simulink model "PMSM_DemoBackup"  (R2020a)
settings: Solver=FixedStepDiscrete  StartTime=0.0  StopTime=Inf  FixedStep=1000e-6  RelTol=1e-3  EnableMultiTasking=on
PreLoadFcn:
  | run('PMSM_Demo_ini.m');
PostLoadFcn:
  | , if any(exist('dsrtsu_mdlpostloadfcn', 'file') ~= 0), dsrtsu_mdlpostloadfcn('Execute', bdroot); end,
InitFcn:
  | , if any(exist('rtifpga_mdlclblib', 'file') ~= 0), rtifpga_mdlclblib('Init', bdroot); end,
undefined symbols (not defined in the file): clock, Const_Id_Fieldweakening, Const_Ld_Stator, Const_Lq_Stator, Const_PolePairs, Const_Psi, Newton, PMSM_Ctrl_Ctrl_mode_SW, PMSM_Ctrl_fRS_Set, PMSM_Ctrl_i_d_Set, PMSM_Ctrl_i_d_Stroke, PMSM_Ctrl_i_q_Set, PMSM_Ctrl_i_q_Stroke, PMSM_Ctrl_Ki_id, PMSM_Ctrl_Ki_iq, PMSM_Ctrl_Ki_n, PMSM_Ctrl_Kp_id, PMSM_Ctrl_Kp_iq, PMSM_Ctrl_Kp_n, PMSM_Ctrl_Limit_iq, PMSM_Ctrl_load_torque, PMSM_Ctrl_n_Limit, PMSM_Ctrl_n_Set, PMSM_Ctrl_n_Stroke, PMSM_Ctrl_Pos_Src, PMSM_Ctrl_TF_Id, PMSM_Ctrl_TF_Iq, PMSM_Ctrl_TF_n, PMSM_Ctrl_theta_offset, PMSM_Ctrl_v_d_Set, PMSM_Ctrl_V_DCLink_Limit, PMSM_Ctrl_v_q_Set, PMSM_Ctrl_Vel_Src, Raphson, rpm_to_rad, s, SW_Fieldweakening, T_PWM
libraries: simulink x37, rti1202lib_adc_class1 x8, dsextras x4, rtiemclib x4, rti1202lib_dio_class1 x3, ASM_ElectricComponents_lib x2, ASM_Utils_lib x1, rti1202lib_base x1
(part 3 of 4)

== system PMSM_DemoBackup/Control/Input/check_inc_valid ==
  note: As long as the encoder has
      | not detected an index signal
      | it's signals are not valid. For this
      | time the hall signals has to be used
  inc_elec_pos : Inport
  hall_pos : Inport  Port=2
  inc_valid : Inport  Port=3
  Switch : Switch  Threshold=0.5
  pos_out : Outport  VectorParamsAs1DForOutWhenUnconnected=off
  wires:
  inc_elec_pos/1 -> Switch/1
  inc_valid/1 -> Switch/2
  Switch/1 -> pos_out/1
  hall_pos/1 -> Switch/3

== system PMSM_DemoBackup/Control/Input/dummy_hall_signals ==
  Ground1 : Ground
  hall_freqbased_vel : Outport  VectorParamsAs1DForOutWhenUnconnected=off
  wires:
  Ground1/1 -> hall_freqbased_vel/1  "hall_freqbased_vel"

== system PMSM_DemoBackup/Control/Input/mech2elec ==
  elec. Angle Offset : Inport
  mech angle : Inport  Port=2
  Constant4 : Constant  Value=360
  Gain3 : Gain  Gain=4
  Math Function : Math  Operator=mod  SignedPower=on  SaturateOnIntegerOverflow=on
  Sum : Sum  Inputs=|++
  elec angle : Outport  VectorParamsAs1DForOutWhenUnconnected=off
  wires:
  elec. Angle Offset/1 -> Sum/1
  Gain3/1 -> Sum/2
  Sum/1 -> Math Function/1
  Math Function/1 -> elec angle/1  "Inc_elec_pos"
  Constant4/1 -> Math Function/2
  mech angle/1 -> Gain3/1

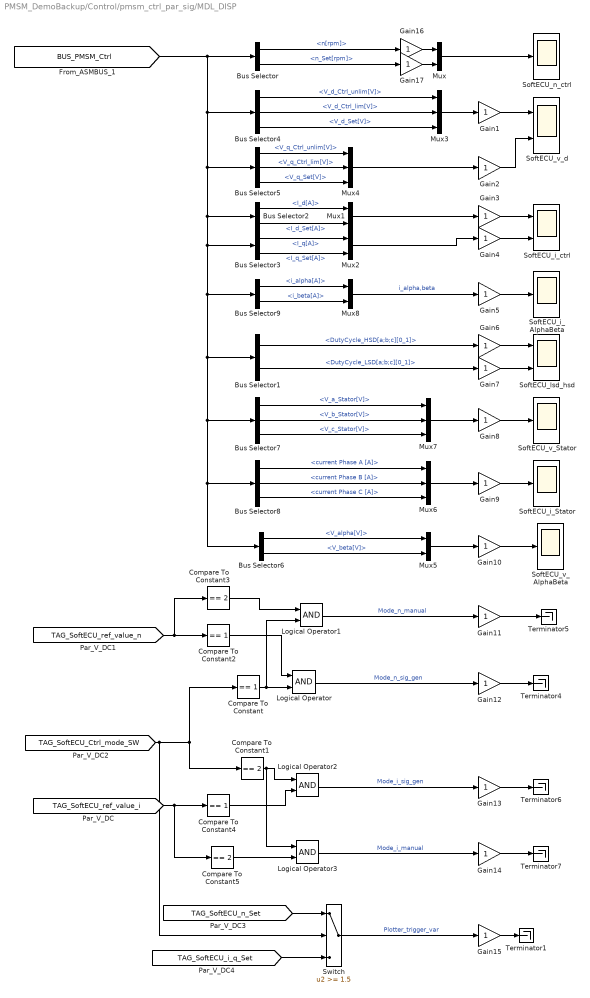
== system PMSM_DemoBackup/Control/pmsm_ctrl_par_sig/MDL_DISP ==
  Bus Selector : BusSelector  OutputSignals=PMSM_Ctrl.PMSM_CONTROLLER.ASMSignalBus_Speed_Controller.n[rpm],PMSM_Ctrl.PMSM_CONTROLLER.ASMSignalBus_Speed_Controller.n_Set[rpm]
  Bus Selector1 : BusSelector  OutputSignals=PMSM_Ctrl.SPACE_VECTOR_MODULATOR.DutyCycle_HSD[a;b;c][0_1],PMSM_Ctrl.SPACE_VECTOR_MODULATOR.DutyCycle_LSD[a;b;c][0_1]
  Bus Selector2 : BusSelector  OutputSignals=PMSM_Ctrl.PMSM_CONTROLLER.ASMSignalBus_Current_Controller.I_d[A],PMSM_Ctrl.PMSM_CONTROLLER.ASMSignalBus_Current_Controller.I_d_Set[A]
  Bus Selector3 : BusSelector  OutputSignals=PMSM_Ctrl.PMSM_CONTROLLER.ASMSignalBus_Current_Controller.I_q[A],PMSM_Ctrl.PMSM_CONTROLLER.ASMSignalBus_Current_Controller.I_q_Set[A]
  Bus Selector4 : BusSelector  OutputSignals=PMSM_Ctrl.PMSM_CONTROLLER.ASMSignalBus_Current_Controller.V_d_Ctrl_unlim[V],PMSM_Ctrl.PMSM_CONTROLLER.ASMSignalBus_Current_Controller.V_d_Ctrl_lim[V],PMSM_Ctrl.PMSM_CONTROLLER.ASMSignalBus_Current_Controller.V_d_Set[V]
  Bus Selector5 : BusSelector  OutputSignals=PMSM_Ctrl.PMSM_CONTROLLER.ASMSignalBus_Current_Controller.V_q_Ctrl_unlim[V],PMSM_Ctrl.PMSM_CONTROLLER.ASMSignalBus_Current_Controller.V_q_Ctrl_lim[V],PMSM_Ctrl.PMSM_CONTROLLER.ASMSignalBus_Current_Controller.V_q_Set[V]
  Bus Selector6 : BusSelector  OutputSignals=PMSM_Ctrl.PMSM_CONTROLLER.V_alpha[V],PMSM_Ctrl.PMSM_CONTROLLER.V_beta[V]
  Bus Selector7 : BusSelector  OutputSignals=PMSM_Ctrl.PMSM_CONTROLLER.v_Stator[a;b;c][V].V_a_Stator[V],PMSM_Ctrl.PMSM_CONTROLLER.v_Stator[a;b;c][V].V_b_Stator[V],PMSM_Ctrl.PMSM_CONTROLLER.v_Stator[a;b;c][V].V_c_Stator[V]
  Bus Selector8 : BusSelector  OutputSignals=PMSM_Ctrl.PMSM_CONTROLLER.i_Stator[a;b;c][A].current Phase A [A],PMSM_Ctrl.PMSM_CONTROLLER.i_Stator[a;b;c][A].current Phase B [A],PMSM_Ctrl.PMSM_CONTROLLER.i_Stator[a;b;c][A].current Phase C [A]
  Bus Selector9 : BusSelector  OutputSignals=PMSM_Ctrl.PMSM_CONTROLLER.ASMSignalBus_Current_Controller.i_alpha[A],PMSM_Ctrl.PMSM_CONTROLLER.ASMSignalBus_Current_Controller.i_beta[A]
  Compare To Constant : simulink/Logic and Bit Operations/Compare To Constant  relop===  const=1  OutDataTypeStr=uint8  ZeroCross=off
  Compare To Constant1 : simulink/Logic and Bit Operations/Compare To Constant  relop===  const=2  OutDataTypeStr=uint8  ZeroCross=off
  Compare To Constant2 : simulink/Logic and Bit Operations/Compare To Constant  relop===  const=1  OutDataTypeStr=uint8  ZeroCross=off
  Compare To Constant3 : simulink/Logic and Bit Operations/Compare To Constant  relop===  const=2  OutDataTypeStr=uint8  ZeroCross=off
  Compare To Constant4 : simulink/Logic and Bit Operations/Compare To Constant  relop===  const=1  OutDataTypeStr=uint8  ZeroCross=off
  Compare To Constant5 : simulink/Logic and Bit Operations/Compare To Constant  relop===  const=2  OutDataTypeStr=uint8  ZeroCross=off
  Gain{1..17} (17 alike) : Gain
  Logical Operator{,1..3} (4 alike) : Logic  AllPortsSameDT=off  OutDataTypeStr=boolean
  Mux{,1..2,5,8} (5 alike) : Mux  Inputs=2
  Mux{3..4,6..7} (4 alike) : Mux  Inputs=3
  SoftECU_i_AlphaBeta : Scope
  SoftECU_i_Stator : Scope
  SoftECU_i_ctrl : Scope  NumInputPorts=2
  SoftECU_lsd_hsd : Scope  NumInputPorts=2
  SoftECU_n_ctrl : Scope
  SoftECU_v_AlphaBeta : Scope
  SoftECU_v_Stator : Scope
  SoftECU_v_d : Scope  NumInputPorts=2
  Switch : Switch  Threshold=1.5
  Terminator{1,4..7} (5 alike) : Terminator
  wires:
  Bus Selector5/3 -> Mux4/3  "<V_q_Set[V]>"
  Bus Selector4/3 -> Mux3/3  "<V_d_Set[V]>"
  Mux2/1 -> Gain4/1
  Mux4/1 -> Gain2/1
  [BUS_PMSM_Ctrl] -> Bus Selector/1, Bus Selector4/1, Bus Selector3/1, Bus Selector7/1, Bus Selector8/1, Bus Selector6/1, Bus Selector1/1, Bus Selector9/1, Bus Selector2/1, Bus Selector5/1
  Bus Selector/1 -> Gain16/1  "<n[rpm]>"
  Bus Selector/2 -> Gain17/1  "<n_Set[rpm]>"
  Bus Selector1/1 -> Gain6/1  "<DutyCycle_HSD[a;b;c][0_1]>"
  Bus Selector1/2 -> Gain7/1  "<DutyCycle_LSD[a;b;c][0_1]>"
  Bus Selector2/1 -> Mux1/1  "<I_d[A]>"
  Bus Selector2/2 -> Mux1/2  "<I_d_Set[A]>"
  Mux1/1 -> Gain3/1
  Bus Selector3/1 -> Mux2/1  "<I_q[A]>"
  Bus Selector3/2 -> Mux2/2  "<I_q_Set[A]>"
  Bus Selector4/1 -> Mux3/1  "<V_d_Ctrl_unlim[V]>"
  Bus Selector4/2 -> Mux3/2  "<V_d_Ctrl_lim[V]>"
  Mux3/1 -> Gain1/1
  Bus Selector5/1 -> Mux4/1  "<V_q_Ctrl_unlim[V]>"
  Bus Selector5/2 -> Mux4/2  "<V_q_Ctrl_lim[V]>"
  Bus Selector6/1 -> Mux5/1  "<V_alpha[V]>"
  Bus Selector6/2 -> Mux5/2  "<V_beta[V]>"
  Mux5/1 -> Gain10/1
  Bus Selector8/1 -> Mux6/1  "<current Phase A [A]>"
  Bus Selector8/2 -> Mux6/2  "<current Phase B [A]>"
  Bus Selector8/3 -> Mux6/3  "<current Phase C [A]>"
  Mux6/1 -> Gain9/1
  Bus Selector7/1 -> Mux7/1  "<V_a_Stator[V]>"
  Bus Selector7/2 -> Mux7/2  "<V_b_Stator[V]>"
  Bus Selector7/3 -> Mux7/3  "<V_c_Stator[V]>"
  Mux7/1 -> Gain8/1
  Bus Selector9/1 -> Mux8/1  "<i_alpha[A]>"
  Bus Selector9/2 -> Mux8/2  "<i_beta[A]>"
  Mux8/1 -> Gain5/1  "i_alpha,beta"
  [TAG_SoftECU_Ctrl_mode_SW] -> Compare To Constant/1, Compare To Constant1/1, Switch/2
  [TAG_SoftECU_ref_value_n] -> Compare To Constant2/1, Compare To Constant3/1
  Compare To Constant/1 -> Logical Operator/2, Logical Operator1/2
  Logical Operator/1 -> Gain12/1  "Mode_n_sig_gen"
  Compare To Constant2/1 -> Logical Operator/1
  Logical Operator1/1 -> Gain11/1  "Mode_n_manual"
  Compare To Constant3/1 -> Logical Operator1/1
  Compare To Constant1/1 -> Logical Operator2/1, Logical Operator3/1
  [TAG_SoftECU_ref_value_i] -> Compare To Constant4/1, Compare To Constant5/1
  Compare To Constant4/1 -> Logical Operator2/2
  Logical Operator2/1 -> Gain13/1  "Mode_i_sig_gen"
  Compare To Constant5/1 -> Logical Operator3/2
  Logical Operator3/1 -> Gain14/1  "Mode_i_manual"
  [TAG_SoftECU_n_Set] -> Switch/1
  [TAG_SoftECU_i_q_Set] -> Switch/3
  Switch/1 -> Gain15/1  "Plotter_trigger_var"
  Mux/1 -> SoftECU_n_ctrl/1
  Gain1/1 -> SoftECU_v_d/1
  Gain2/1 -> SoftECU_v_d/2
  Gain3/1 -> SoftECU_i_ctrl/1
  Gain4/1 -> SoftECU_i_ctrl/2
  Gain5/1 -> SoftECU_i_AlphaBeta/1
  Gain6/1 -> SoftECU_lsd_hsd/1
  Gain7/1 -> SoftECU_lsd_hsd/2
  Gain8/1 -> SoftECU_v_Stator/1
  Gain9/1 -> SoftECU_i_Stator/1
  Gain10/1 -> SoftECU_v_AlphaBeta/1
  Gain11/1 -> Terminator5/1
  Gain12/1 -> Terminator4/1
  Gain13/1 -> Terminator6/1
  Gain14/1 -> Terminator7/1
  Gain15/1 -> Terminator1/1
  Gain16/1 -> Mux/1
  Gain17/1 -> Mux/2

== system PMSM_DemoBackup/Control/pmsm_ctrl_par_sig/MDL_DISP_INPUT ==
  Bus Selector2 : BusSelector  OutputSignals=PMSM_in.Hall_Signals.hall_elec_pos,PMSM_in.Hall_Signals.hall_freqbased_vel,PMSM_in.Hall_Signals.hall_signals
  Bus Selector3 : BusSelector  OutputSignals=PMSM_in.ADC_Voltages
  Bus Selector4 : BusSelector  OutputSignals=PMSM_in.Inc_Signals.Inc_mech_pos,PMSM_in.Inc_Signals.Inc_elec_pos,PMSM_in.Inc_Signals.inc_derivative_vel
  Mux1 : Mux  Inputs=3
  Mux2 : Mux  Inputs=1
  Mux3 : Mux  Inputs=3
  Terminator1 : Terminator
  Terminator2 : Terminator
  Terminator3 : Terminator
  wires:
  [BUS_Inputs] -> Bus Selector4/1, Bus Selector2/1, Bus Selector3/1
  Mux2/1 -> Terminator3/1
  Bus Selector2/1 -> Mux1/1  "<hall_elec_pos>"
  Mux1/1 -> Terminator2/1
  Bus Selector3/1 -> Mux2/1  "<ADC_Voltages>"
  Bus Selector2/2 -> Mux1/2  "<hall_freqbased_vel>"
  Bus Selector4/1 -> Mux3/1  "<Inc_mech_pos>"
  Bus Selector4/2 -> Mux3/2  "<Inc_elec_pos>"
  Mux3/1 -> Terminator1/1
  Bus Selector2/3 -> Mux1/3  "<hall_signals>"
  Bus Selector4/3 -> Mux3/3  "<inc_derivative_vel>"

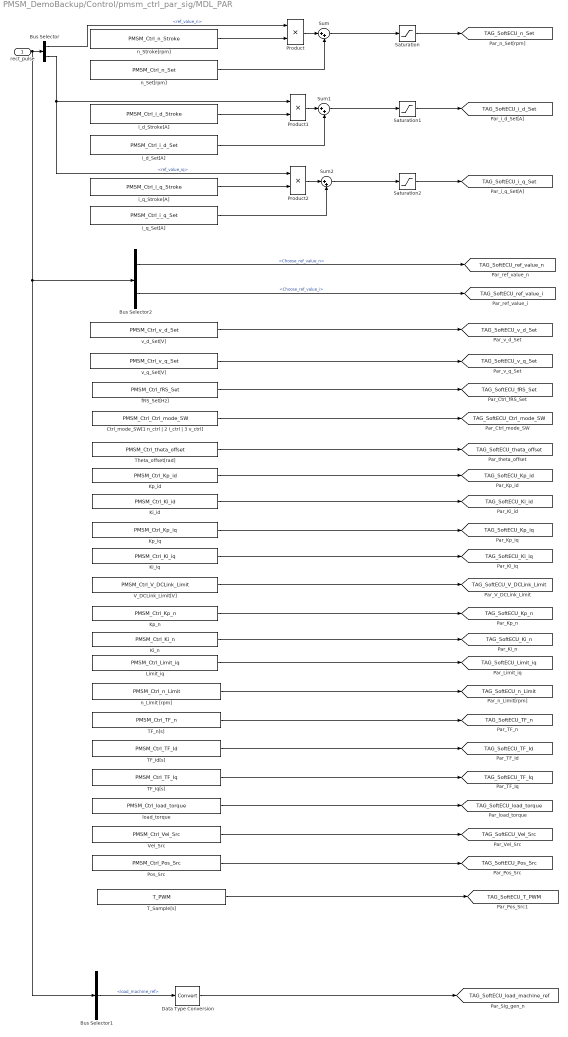
== system PMSM_DemoBackup/Control/pmsm_ctrl_par_sig/MDL_PAR ==
  rect_pulse : Inport
  Bus Selector : BusSelector  OutputSignals=ref_value_n,ref_value_iq
  Bus Selector1 : BusSelector  OutputSignals=load_machine_ref
  Bus Selector2 : BusSelector  OutputSignals=Choose_ref_value_n,Choose_ref_value_i
  Ctrl_mode_SW[1 n_ctrl | 2 i_ctrl | 3 v_ctrl] : Constant  Value=PMSM_Ctrl_Ctrl_mode_SW
  Data Type Conversion : DataTypeConversion
  Ki_id : Constant  Value=PMSM_Ctrl_Ki_id
  Ki_iq : Constant  Value=PMSM_Ctrl_Ki_iq
  Ki_n : Constant  Value=PMSM_Ctrl_Ki_n
  Kp_id : Constant  Value=PMSM_Ctrl_Kp_id
  Kp_iq : Constant  Value=PMSM_Ctrl_Kp_iq
  Kp_n : Constant  Value=PMSM_Ctrl_Kp_n
  Limit_iq : Constant  Value=PMSM_Ctrl_Limit_iq
  Pos_Src : Constant  Value=PMSM_Ctrl_Pos_Src
  Product : Product  RndMeth=Zero
  Product1 : Product  RndMeth=Zero
  Product2 : Product  RndMeth=Zero
  Saturation : Saturate  UpperLimit=1200  LowerLimit=-1200
  Saturation1 : Saturate  UpperLimit=6  LowerLimit=-6
  Saturation2 : Saturate  UpperLimit=6  LowerLimit=-6
  Sum : Sum  Inputs=|++
  Sum1 : Sum  Inputs=|++
  Sum2 : Sum  Inputs=|++
  TF_Id[s] : Constant  Value=PMSM_Ctrl_TF_Id
  TF_Iq[s] : Constant  Value=PMSM_Ctrl_TF_Iq
  TF_n[s] : Constant  Value=PMSM_Ctrl_TF_n
  T_Sample[s] : Constant  Value=T_PWM
  Theta_offset[rad] : Constant  Value=PMSM_Ctrl_theta_offset
  V_DCLink_Limit[V] : Constant  Value=PMSM_Ctrl_V_DCLink_Limit
  Vel_Src : Constant  Value=PMSM_Ctrl_Vel_Src
  fRS_Set[Hz] : Constant  Value=PMSM_Ctrl_fRS_Set
  i_d_Set[A] : Constant  Value=PMSM_Ctrl_i_d_Set
  i_d_Stroke[A] : Constant  Value=PMSM_Ctrl_i_d_Stroke
  i_q_Set[A] : Constant  Value=PMSM_Ctrl_i_q_Set
  i_q_Stroke[A] : Constant  Value=PMSM_Ctrl_i_q_Stroke
  load_torque : Constant  Value=PMSM_Ctrl_load_torque
  n_Limit [rpm] : Constant  Value=PMSM_Ctrl_n_Limit
  n_Set[rpm] : Constant  Value=PMSM_Ctrl_n_Set
  n_Stroke[rpm] : Constant  Value=PMSM_Ctrl_n_Stroke
  v_d_Set[V] : Constant  Value=PMSM_Ctrl_v_d_Set
  v_q_Set[V] : Constant  Value=PMSM_Ctrl_v_q_Set
  tag scope: TAG_SoftECU_Ctrl_mode_SW=global, TAG_SoftECU_Ki_id=global, TAG_SoftECU_Ki_iq=global, TAG_SoftECU_Ki_n=global, TAG_SoftECU_Kp_id=global, TAG_SoftECU_Kp_iq=global, TAG_SoftECU_Kp_n=global, TAG_SoftECU_Limit_iq=global, TAG_SoftECU_Pos_Src=global, TAG_SoftECU_TF_Id=global, TAG_SoftECU_TF_Iq=global, TAG_SoftECU_TF_n=global, TAG_SoftECU_T_PWM=global, TAG_SoftECU_V_DCLink_Limit=global, TAG_SoftECU_Vel_Src=global, TAG_SoftECU_fRS_Set=global, TAG_SoftECU_i_d_Set=global, TAG_SoftECU_i_q_Set=global, TAG_SoftECU_load_machine_ref=global, TAG_SoftECU_load_torque=global, TAG_SoftECU_n_Limit=global, TAG_SoftECU_n_Set=global, TAG_SoftECU_ref_value_i=global, TAG_SoftECU_ref_value_n=global, TAG_SoftECU_theta_offset=global, TAG_SoftECU_v_d_Set=global, TAG_SoftECU_v_q_Set=global
  wires:
  Limit_iq/1 -> [TAG_SoftECU_Limit_iq]
  Ki_n/1 -> [TAG_SoftECU_Ki_n]
  Kp_n/1 -> [TAG_SoftECU_Kp_n]
  V_DCLink_Limit[V]/1 -> [TAG_SoftECU_V_DCLink_Limit]
  Ki_iq/1 -> [TAG_SoftECU_Ki_iq]
  Kp_iq/1 -> [TAG_SoftECU_Kp_iq]
  Ki_id/1 -> [TAG_SoftECU_Ki_id]
  Kp_id/1 -> [TAG_SoftECU_Kp_id]
  Theta_offset[rad]/1 -> [TAG_SoftECU_theta_offset]
  v_d_Set[V]/1 -> [TAG_SoftECU_v_d_Set]
  Ctrl_mode_SW[1 n_ctrl | 2 i_ctrl | 3 v_ctrl]/1 -> [TAG_SoftECU_Ctrl_mode_SW]
  fRS_Set[Hz]/1 -> [TAG_SoftECU_fRS_Set]
  v_q_Set[V]/1 -> [TAG_SoftECU_v_q_Set]
  n_Limit [rpm]/1 -> [TAG_SoftECU_n_Limit]
  TF_n[s]/1 -> [TAG_SoftECU_TF_n]
  TF_Id[s]/1 -> [TAG_SoftECU_TF_Id]
  TF_Iq[s]/1 -> [TAG_SoftECU_TF_Iq]
  load_torque/1 -> [TAG_SoftECU_load_torque]
  Sum/1 -> Saturation/1
  Product/1 -> Sum/1
  Product1/1 -> Sum1/1
  Sum1/1 -> Saturation1/1
  Product2/1 -> Sum2/1
  Sum2/1 -> Saturation2/1
  n_Set[rpm]/1 -> Sum/2
  i_d_Set[A]/1 -> Sum1/2
  i_q_Set[A]/1 -> Sum2/2
  n_Stroke[rpm]/1 -> Product/2
  i_d_Stroke[A]/1 -> Product1/2
  i_q_Stroke[A]/1 -> Product2/2
  Vel_Src/1 -> [TAG_SoftECU_Vel_Src]
  Pos_Src/1 -> [TAG_SoftECU_Pos_Src]
  T_Sample[s]/1 -> [TAG_SoftECU_T_PWM]
  Saturation/1 -> [TAG_SoftECU_n_Set]
  Saturation1/1 -> [TAG_SoftECU_i_d_Set]
  Saturation2/1 -> [TAG_SoftECU_i_q_Set]
  rect_pulse/1 -> Bus Selector/1, Bus Selector1/1, Bus Selector2/1
  Bus Selector/1 -> Product/1  "<ref_value_n>"
  Bus Selector/2 -> Product1/1, Product2/1  "<ref_value_iq>"
  Bus Selector1/1 -> Data Type Conversion/1  "<load_machine_ref>"
  Bus Selector2/1 -> [TAG_SoftECU_ref_value_n]  "<Choose_ref_value_n>"
  Bus Selector2/2 -> [TAG_SoftECU_ref_value_i]  "<Choose_ref_value_i>"
  Data Type Conversion/1 -> [TAG_SoftECU_load_machine_ref]

== system PMSM_DemoBackup/RTI Data/RTI Data Store/RTI Data Store ==
  RTI Data Store : Subsystem  mask(RTI_DATA_STORE){}
      mask help:
      | RTI Data Store Block. This block is used by RTI to store internal model dependent data. Deleting this block will result in data loss.
      |
      | NEVER DELETE, COPY, OR MODIFY THIS BLOCK!
      mask Help:
      | RTI Data Store Block. This block is used by RTI to store internal model dependent data. Deleting this block will result in data loss.
      | 
      | NEVER DELETE, COPY, OR MODIFY THIS BLOCK!
      mask Display: text(0.5, 0.5, ' ', 'HorizontalAlignment', 'center');

== system PMSM_DemoBackup/Control/Control_load_machine/duty_cycle_2_torque/duty_cycle_2_voltage ==
  In_duty_cycle[0..1] : Inport
  Bus Selector : BusSelector  OutputSignals=ADC_Voltages.Battery_Voltage[V]
  Divide : Product  Inputs=**
  Saturation1 : Saturate  UpperLimit=1  LowerLimit=0
  Out_duty_voltage[V] : Outport  VectorParamsAs1DForOutWhenUnconnected=off
  wires:
  Divide/1 -> Out_duty_voltage[V]/1
  In_duty_cycle[0..1]/1 -> Saturation1/1
  Bus Selector/1 -> Divide/2  "<Battery_Voltage[V]>"
  [BUS_PMSM_IN] -> Bus Selector/1
  Saturation1/1 -> Divide/1

== system PMSM_DemoBackup/Control/Control_load_machine/torque_2_duty_cycle/voltage_2_duty_cycle ==
  In_voltage[V] : Inport
  Bus Selector : BusSelector  OutputSignals=ADC_Voltages.Battery_Voltage[V]
  Divide : Product  Inputs=*/
  Saturation : Saturate  UpperLimit=1  LowerLimit=0
  Out_duty_cycle : Outport  VectorParamsAs1DForOutWhenUnconnected=off
  wires:
  Divide/1 -> Saturation/1
  In_voltage[V]/1 -> Divide/1
  Saturation/1 -> Out_duty_cycle/1
  Bus Selector/1 -> Divide/2  "<Battery_Voltage[V]>"
  [BUS_PMSM_IN] -> Bus Selector/1

== system PMSM_DemoBackup/Control/Control_load_machine/torque_2_duty_cycle1/voltage_2_duty_cycle ==
  In_voltage[V] : Inport
  Bus Selector : BusSelector  OutputSignals=ADC_Voltages.Battery_Voltage[V]
  Divide : Product  Inputs=*/
  Saturation : Saturate  UpperLimit=1  LowerLimit=0
  Out_duty_cycle[0..1] : Outport  VectorParamsAs1DForOutWhenUnconnected=off
  wires:
  [BUS_PMSM_IN] -> Bus Selector/1
  Bus Selector/1 -> Divide/2  "<Battery_Voltage[V]>"
  Saturation/1 -> Out_duty_cycle[0..1]/1
  In_voltage[V]/1 -> Divide/1
  Divide/1 -> Saturation/1

== system PMSM_DemoBackup/Control/Controller/PMSM_CONTROLLER/5x_mean_value ==
  n[rpm] : Inport
  Gain : Gain  Gain=1/5
  Memory{,1..3} (4 alike) : Memory  InheritSampleTime=on
  Sum : Sum  Inputs=+++++
  n_mean[rpm] : Outport  VectorParamsAs1DForOutWhenUnconnected=off
  wires:
  n[rpm]/1 -> Sum/1, Memory/1
  Memory/1 -> Sum/2, Memory1/1
  Memory1/1 -> Sum/3, Memory2/1
  Memory2/1 -> Sum/4, Memory3/1
  Memory3/1 -> Sum/5
  Sum/1 -> Gain/1
  Gain/1 -> n_mean[rpm]/1

== system PMSM_DemoBackup/Control/Controller/PMSM_CONTROLLER/SignalCollector ==
  SignalBus_Speed_Controller : Inport
  V_DCLink[V] : Inport  Port=2
  i_Stator[a;b;c][A] : Inport  Port=3
  SignalBus_Current_Controller : Inport  Port=4
  V_d[V] : Inport  Port=5
  V_q[V] : Inport  Port=6
  V_alpha[V] : Inport  Port=7
  V_beta[V] : Inport  Port=8
  v_Stator[a;b;c][V] : Inport  Port=9
  Bus Creator : BusCreator  Inputs=9
  SignalBus : Outport  VectorParamsAs1DForOutWhenUnconnected=off
  wires:
  SignalBus_Current_Controller/1 -> Bus Creator/2  "ASMSignalBus_Current_Controller"
  SignalBus_Speed_Controller/1 -> Bus Creator/1  "ASMSignalBus_Speed_Controller"
  V_q[V]/1 -> Bus Creator/7  "V_q_Set[V]"
  V_d[V]/1 -> Bus Creator/6  "V_d_Set[V]"
  Bus Creator/1 -> SignalBus/1  "PMSM_CONTROLLER"
  V_DCLink[V]/1 -> Bus Creator/5  "V_DCLink[V]"
  i_Stator[a;b;c][A]/1 -> Bus Creator/3  "i_Stator[a;b;c][A]"
  v_Stator[a;b;c][V]/1 -> Bus Creator/4  "v_Stator[a;b;c][V]"
  V_alpha[V]/1 -> Bus Creator/8  "V_alpha[V]"
  V_beta[V]/1 -> Bus Creator/9  "V_beta[V]"

== system PMSM_DemoBackup/Control/Controller/PMSM_CONTROLLER/Trigger_250us ==
  Counter Limited : simulink/Sources/Counter Limited  uplimit=4  tsamp=-1
  Lookup Table : Lookup_n-D  NumberOfTableDimensions=1  BreakpointsForDimension1=[0,1,2,3,4]  Table=[1,0,0,0,0]  ExtrapMethod=Clip  InputSameDT=on
  trigger : Outport  VectorParamsAs1DForOutWhenUnconnected=off
  wires:
  Counter Limited/1 -> Lookup Table/1
  Lookup Table/1 -> trigger/1

== system PMSM_DemoBackup/Control/Controller/PMSM_CONTROLLER/angle_calculation ==
  n[rpm] : Inport
  eps [rad] : Inport  Port=2
  eps_offset[rad] : Inport  Port=3
  T_Sample[s] : Inport  Port=4
  Const_PolePair[] : Constant  Value=Const_PolePair
  Lim[0...2*pi] : Subsystem
  Product1 : Product  RndMeth=Zero
  Product2 : Product  RndMeth=Zero
  Sum : Sum  Inputs=|++
  Terminator : Terminator
  toRad|s : Gain  Gain=pi/30  SaturateOnIntegerOverflow=on  OutDataTypeStr=Inherit: Same as input  ParamDataTypeStr=Inherit: Same as input
  eps[rad] : Outport  VectorParamsAs1DForOutWhenUnconnected=off
  omega_el[rad|s] : Outport  Port=2  VectorParamsAs1DForOutWhenUnconnected=off
  eps_komp[rad] : Outport  Port=3  VectorParamsAs1DForOutWhenUnconnected=off
  wires:
  n[rpm]/1 -> Product2/1
  T_Sample[s]/1 -> Product1/1
  Product1/1 -> Terminator/1
  toRad|s/1 -> Product1/2, omega_el[rad|s]/1
  Product2/1 -> toRad|s/1
  Const_PolePair[]/1 -> Product2/2
  Lim[0...2*pi]/1(theta_lim) -> eps[rad]/1, eps_komp[rad]/1
  eps [rad]/1 -> Sum/1
  Sum/1 -> Lim[0...2*pi]/1(theta_unlim)
  eps_offset[rad]/1 -> Sum/2

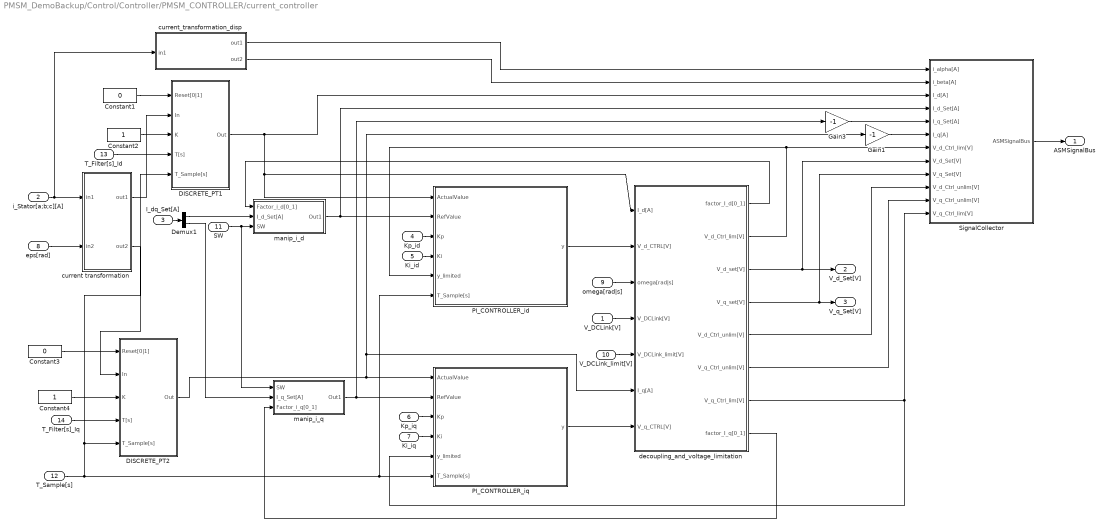
== system PMSM_DemoBackup/Control/Controller/PMSM_CONTROLLER/current_controller ==
  V_DCLink[V] : Inport
  i_Stator[a;b;c][A] : Inport  Port=2
  I_dq_Set[A] : Inport  Port=3
  Kp_id : Inport  Port=4
  Ki_id : Inport  Port=5
  Kp_iq : Inport  Port=6
  Ki_iq : Inport  Port=7
  eps[rad] : Inport  Port=8
  omega[rad|s] : Inport  Port=9
  V_DCLink_limit[V] : Inport  Port=10
  SW : Inport  Port=11
  T_Sample[s] : Inport  Port=12
  T_Filter[s]_Id : Inport  Port=13
  T_Filter[s]_Iq : Inport  Port=14
  Constant1 : Constant  Value=0
  Constant2 : Constant
  Constant3 : Constant  Value=0
  Constant4 : Constant
  DISCRETE_PT1 : Subsystem  mask(DISCRETE_PT1){upper_limit_int=struct('v', 1e300), lower_limit_int=struct('v', -1e300), ASMProperties=struct('Name','DISCRETE_PT1','Version','1.0','Library','ASM_ElectricComponents_lib')}
      mask prompts: upper_limit_int "upper limit (Integrator)"; lower_limit_int "lower limit (Integrator)"
      mask help: (c) Copyright 2007, dSPACE GmbH. All rights reserved.
      mask Help: eval(['asm_modelhelp(gcbh)'])
  DISCRETE_PT2 : Subsystem  mask(DISCRETE_PT1){upper_limit_int=struct('v', 1e300), lower_limit_int=struct('v', -1e300), ASMProperties=struct('Name','DISCRETE_PT1','Version','1.0','Library','ASM_ElectricComponents_lib')}
      mask prompts: upper_limit_int "upper limit (Integrator)"; lower_limit_int "lower limit (Integrator)"
      mask help: (c) Copyright 2007, dSPACE GmbH. All rights reserved.
      mask Help: eval(['asm_modelhelp(gcbh)'])
  Demux1 : Demux  Outputs=2
  Gain1 : Gain  Gain=-1
  Gain3 : Gain  Gain=-1
  PI_CONTROLLER_id : Subsystem  mask(PI_CONTROLLER_EXT_SATURATION){ASMProperties=struct('Name','PI_CONTROLLER_EXT_SATURATION','Version','1.0','Library','ASM_ElectricComponents_lib')}
      mask help: (c) Copyright 2007, dSPACE GmbH. All rights reserved.
  PI_CONTROLLER_iq : Subsystem  mask(PI_CONTROLLER_EXT_SATURATION){ASMProperties=struct('Name','PI_CONTROLLER_EXT_SATURATION','Version','1.0','Library','ASM_ElectricComponents_lib')}
      mask help: (c) Copyright 2007, dSPACE GmbH. All rights reserved.
  SignalCollector : Subsystem
  current transformation : Subsystem  Description=version  mask(ASM_EC_TRANSFORMATION){transformation=abc            -> d/q              (clarke and park transformation), compin=off, compout=on, zerocomp=off, interm=off, cossinvector=off, powrefframe=off, transffactor=1, transffactor_zero=1, ASMProperties=struct('Name','asm_ec_transformation','Version','1.0','Library','ASM_ElectricComponents_lib')}
      mask prompts: compin "Component wise input"; compout "Component wise output"; zerocomp "Zero component"; interm "Intermediat values"; cossinvector "Cos/Sin vector input"; powrefframe "Power-invariant transformation"
      mask help:
      | Clarke and/or Park transformation for three phase electric system.
      |
      | (c) Copyright 2007, dSPACE GmbH. All rights reserved.
      mask init:
      | %asm_ec_clarkparktrans('DYNATRANSF_Config',gcb);
      settings: AttributesFormatString=park/clark transformation
      mask Help: eval(['asm_modelhelp(gcbh)'])
      mask TypeOptions transformation: abc             -> alpha/beta  (clarke transformation) | alpha/beta -> abc              (inverse clarke transformation) | alpha/beta -> d/q              (park transformation) | d/q             -> alpha/beta  (inverse park transformation) | abc            -> d/q              (clarke and park transformation) | d/q            -> abc              (inverse clarke and park transformation)
      mask Callback transformation: asm_ec_clarkparktrans('DYNATRANSF_ConfigDisp',gcb);
      mask Display: plot([1 0],[1 0]);port_label('input',1,'[3]');port_label('input',2,'eps (rad)');port_label('output',1,'d');port_label('output',2,'q');text(0.042857,0.94898,'a,b,c');text(0.89286,0.05102,'');
  current_transformation_disp : Subsystem  Description=version  mask(ASM_EC_TRANSFORMATION){transformation=abc             -> alpha/beta  (clarke transformation), compin=off, compout=on, zerocomp=off, interm=off, cossinvector=off, powrefframe=off, transffactor=1, transffactor_zero=1, ASMProperties=struct('Name','ASM_EC_TRANSFORMATION','Version','1.0','Library','ASM_ElectricComponents_lib')}
      mask prompts: compin "Component wise input"; compout "Component wise output"; zerocomp "Zero component"; interm "Intermediat values"; cossinvector "Cos/Sin vector input"; powrefframe "Power-invariant transformation"
      mask help:
      | Clarke and/or Park transformation for three phase electric system.
      |
      | (c) Copyright 2007, dSPACE GmbH. All rights reserved.
      mask init:
      | %asm_ec_clarkparktrans('DYNATRANSF_Config',gcb);
      settings: AttributesFormatString=clark transformation
      mask Help: eval(['asm_modelhelp(gcbh)'])
      mask TypeOptions transformation: abc             -> alpha/beta  (clarke transformation) | alpha/beta -> abc              (inverse clarke transformation) | alpha/beta -> d/q              (park transformation) | d/q             -> alpha/beta  (inverse park transformation) | abc            -> d/q              (clarke and park transformation) | d/q            -> abc              (inverse clarke and park transformation)
      mask Callback transformation: asm_ec_clarkparktrans('DYNATRANSF_ConfigDisp',gcb);
      mask Display: plot([1 0],[1 0]);port_label('input',1,'[3]');port_label('output',1,'alpha');port_label('output',2,'beta');text(0.022222,0.85849,'a,b,c');text(0.94444,0.14151,'');
  decoupling_and_voltage_limitation : Subsystem
  manip_i_d : Subsystem
  manip_i_q : Subsystem
  ASMSignalBus : Outport  VectorParamsAs1DForOutWhenUnconnected=off
  " V_d_Set[V]" : Outport  Port=2  VectorParamsAs1DForOutWhenUnconnected=off
  " V_q_Set[V]" : Outport  Port=3  VectorParamsAs1DForOutWhenUnconnected=off
  wires:
  eps[rad]/1 -> current transformation/2(in2)
  i_Stator[a;b;c][A]/1 -> current transformation/1(in1), current_transformation_disp/1(in1)
  SW/1 -> manip_i_q/1(SW), manip_i_d/3(SW)
  decoupling_and_voltage_limitation/1(factor_I_d[0_1]) -> manip_i_d/1(Factor_i_d[0_1])
  decoupling_and_voltage_limitation/8(factor_I_q[0_1]) -> manip_i_q/3(Factor_i_q[0_1])
  T_Sample[s]/1 -> PI_CONTROLLER_id/6(T_Sample[s]), PI_CONTROLLER_iq/6(T_Sample[s]), DISCRETE_PT1/5(T_Sample[s]), DISCRETE_PT2/5(T_Sample[s])
  Demux1/1 -> manip_i_d/2(I_d_Set[A])
  Demux1/2 -> manip_i_q/2(I_q_Set[A])
  Ki_iq/1 -> PI_CONTROLLER_iq/4(Ki)
  Kp_iq/1 -> PI_CONTROLLER_iq/3(Kp)
  Ki_id/1 -> PI_CONTROLLER_id/4(Ki)
  Kp_id/1 -> PI_CONTROLLER_id/3(Kp)
  manip_i_q/1(Out1) -> PI_CONTROLLER_iq/2(RefValue), Gain3/1
  I_dq_Set[A]/1 -> Demux1/1
  decoupling_and_voltage_limitation/6(V_q_Ctrl_unlim[V]) -> SignalCollector/11(V_q_Ctrl_unlim[V])
  decoupling_and_voltage_limitation/5(V_d_Ctrl_unlim[V]) -> SignalCollector/10(V_d_Ctrl_unlim[V])
  SignalCollector/1(ASMSignalBus) -> ASMSignalBus/1
  decoupling_and_voltage_limitation/2(V_d_Ctrl_lim[V]) -> PI_CONTROLLER_id/5(y_limited), SignalCollector/7(V_d_Ctrl_lim[V])
  decoupling_and_voltage_limitation/7(V_q_Ctrl_lim[V]) -> PI_CONTROLLER_iq/5(y_limited), SignalCollector/12(V_q_Ctrl_lim[V])
  V_DCLink[V]/1 -> decoupling_and_voltage_limitation/4(V_DCLink[V])
  manip_i_d/1(Out1) -> SignalCollector/4(I_d_Set[A]), PI_CONTROLLER_id/2(RefValue)
  omega[rad|s]/1 -> decoupling_and_voltage_limitation/3(omega[rad|s])
  PI_CONTROLLER_iq/1(y) -> decoupling_and_voltage_limitation/7(V_q_CTRL[V])
  decoupling_and_voltage_limitation/4(V_q_set[V]) -> " V_q_Set[V]"/1, SignalCollector/9(V_q_Set[V])
  decoupling_and_voltage_limitation/3(V_d_set[V]) -> " V_d_Set[V]"/1, SignalCollector/8(V_d_Set[V])
  PI_CONTROLLER_id/1(y) -> decoupling_and_voltage_limitation/2(V_d_CTRL[V])
  V_DCLink_limit[V]/1 -> decoupling_and_voltage_limitation/5(V_DCLink_limit[V])
  T_Filter[s]_Iq/1 -> DISCRETE_PT2/4(T[s])
  Constant3/1 -> DISCRETE_PT2/1(Reset[0|1])
  Constant4/1 -> DISCRETE_PT2/3(K)
  current transformation/2(out2) -> DISCRETE_PT2/2(In)
  DISCRETE_PT2/1(Out) -> PI_CONTROLLER_iq/1(ActualValue), decoupling_and_voltage_limitation/6(I_q[A]), Gain1/1
  DISCRETE_PT1/1(Out) -> SignalCollector/3(I_d[A]), PI_CONTROLLER_id/1(ActualValue), decoupling_and_voltage_limitation/1(I_d[A])
  current transformation/1(out1) -> DISCRETE_PT1/2(In)
  Constant1/1 -> DISCRETE_PT1/1(Reset[0|1])
  Constant2/1 -> DISCRETE_PT1/3(K)
  T_Filter[s]_Id/1 -> DISCRETE_PT1/4(T[s])
  Gain3/1 -> SignalCollector/5(I_q_Set[A])
  Gain1/1 -> SignalCollector/6(I_q[A])
  current_transformation_disp/1(out1) -> SignalCollector/1(i_alpha[A])
  current_transformation_disp/2(out2) -> SignalCollector/2(i_beta[A])

== system PMSM_DemoBackup/Control/Controller/PMSM_CONTROLLER/i_set_source_SW ==
  I_d_Set_2 : Inport
  I_q_Set_2 : Inport  Port=2
  I_q_Set_1 : Inport  Port=3
  Id_Limit : Inport  Port=4
  Iq_Limit : Inport  Port=5
  SW : Inport  Port=6
  Const_Id_Fieldweakening[A] : Constant  Value=Const_Id_Fieldweakening
  Demux : Demux  Outputs=2
  Gain3 : Gain  Gain=-1
  Limit_id_Set : Subsystem
      mask Display: plot([0.15 0.85],[.5 .5],[.5 .5],[0.05 0.95],0.15+0.7*[0 .25 .75 1],0.05+0.9*[.25 .25 .75 .75]);
  Limit_iq_Set : Subsystem
      mask Display: plot([0.15 0.85],[.5 .5],[.5 .5],[0.05 0.95],0.15+0.7*[0 .25 .75 1],0.05+0.9*[.25 .25 .75 .75]);
  Multiport Switch : MultiPortSwitch
  Mux{,1..3} (4 alike) : Mux  Inputs=2
  zero : Constant  Value=0
  I_dq_Set : Outport  VectorParamsAs1DForOutWhenUnconnected=off
  wires:
  zero/1 -> Mux3/2, Mux3/1
  Mux3/1 -> Multiport Switch/4
  Mux2/1 -> Multiport Switch/3
  Mux1/1 -> Multiport Switch/2
  Mux/1 -> I_dq_Set/1
  Iq_Limit/1 -> Limit_iq_Set/2(In2)
  Id_Limit/1 -> Limit_id_Set/2(In2)
  Limit_id_Set/1(Out1) -> Mux/1
  Demux/1 -> Limit_id_Set/1(In1)
  Limit_iq_Set/1(Out1) -> Mux/2
  Demux/2 -> Limit_iq_Set/1(In1)
  Multiport Switch/1 -> Demux/1
  I_q_Set_1/1 -> Mux1/2
  SW/1 -> Multiport Switch/1
  I_d_Set_2/1 -> Mux2/1
  I_q_Set_2/1 -> Gain3/1
  Const_Id_Fieldweakening[A]/1 -> Mux1/1
  Gain3/1 -> Mux2/2

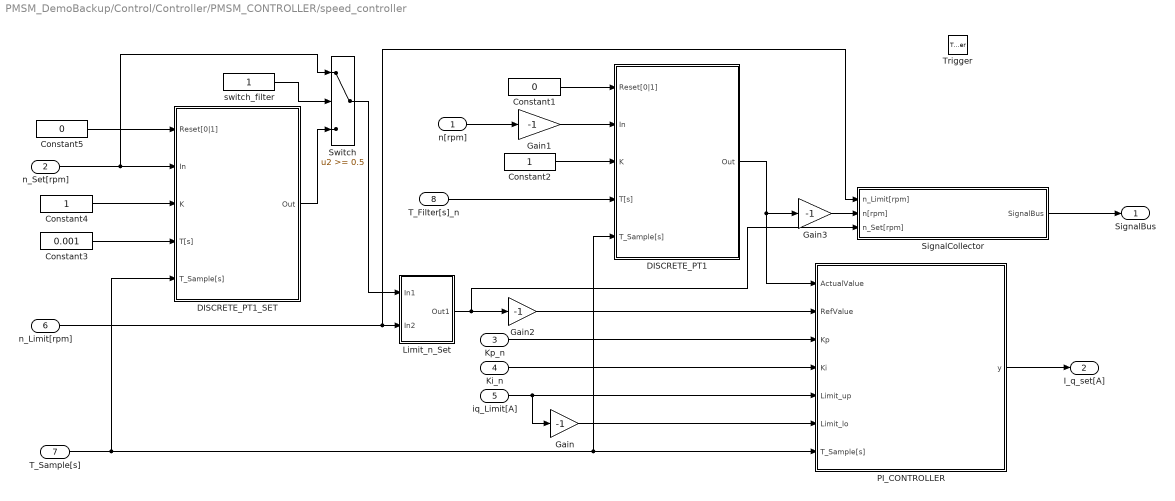
== system PMSM_DemoBackup/Control/Controller/PMSM_CONTROLLER/speed_controller ==
  n[rpm] : Inport
  n_Set[rpm] : Inport  Port=2
  Kp_n : Inport  Port=3
  Ki_n : Inport  Port=4
  iq_Limit[A] : Inport  Port=5
  n_Limit[rpm] : Inport  Port=6
  T_Sample[s] : Inport  Port=7
  T_Filter[s]_n : Inport  Port=8
  Trigger : TriggerPort  VariantControl=Variant
  Constant1 : Constant  Value=0
  Constant2 : Constant
  Constant3 : Constant  Value=0.001
  Constant4 : Constant
  Constant5 : Constant  Value=0
  DISCRETE_PT1 : Subsystem  mask(DISCRETE_PT1){upper_limit_int=struct('v',1e300), lower_limit_int=struct('v', -1e300), ASMProperties=struct('Name','DISCRETE_PT1','Version','1.0','Library','ASM_ElectricComponents_lib')}
      mask prompts: upper_limit_int "upper limit (Integrator)"; lower_limit_int "lower limit (Integrator)"
      mask help: (c) Copyright 2007, dSPACE GmbH. All rights reserved.
      mask Help: eval(['asm_modelhelp(gcbh)'])
  DISCRETE_PT1_SET : Subsystem  mask(DISCRETE_PT1){upper_limit_int=struct('v', 1e300), lower_limit_int=struct('v', -1e300), ASMProperties=struct('Name','DISCRETE_PT1','Version','1.0','Library','ASM_ElectricComponents_lib')}
      mask prompts: upper_limit_int "upper limit (Integrator)"; lower_limit_int "lower limit (Integrator)"
      mask help: (c) Copyright 2007, dSPACE GmbH. All rights reserved.
      mask Help: eval(['asm_modelhelp(gcbh)'])
  Gain{,1..3} (4 alike) : Gain  Gain=-1
  Limit_n_Set : Subsystem
      mask Display: plot([0.15 0.85],[.5 .5],[.5 .5],[0.05 0.95],0.15+0.7*[0 .25 .75 1],0.05+0.9*[.25 .25 .75 .75]);
  PI_CONTROLLER : Subsystem  mask(PI_CONTROLLER){ASMProperties=struct('Name','PI_CONTROLLER','Version','1.0','Library','ASM_ElectricComponents_lib')}
      mask help: (c) Copyright 2007, dSPACE GmbH. All rights reserved.
  SignalCollector : Subsystem
  Switch : Switch  Threshold=0.5
  switch_filter : Constant
  SignalBus : Outport  VectorParamsAs1DForOutWhenUnconnected=off
  I_q_set[A] : Outport  Port=2  VectorParamsAs1DForOutWhenUnconnected=off
  wires:
  SignalCollector/1(SignalBus) -> SignalBus/1
  PI_CONTROLLER/1(y) -> I_q_set[A]/1
  Kp_n/1 -> PI_CONTROLLER/3(Kp)
  Ki_n/1 -> PI_CONTROLLER/4(Ki)
  iq_Limit[A]/1 -> PI_CONTROLLER/5(Limit_up), Gain/1
  Gain/1 -> PI_CONTROLLER/6(Limit_lo)
  T_Sample[s]/1 -> PI_CONTROLLER/7(T_Sample[s]), DISCRETE_PT1/5(T_Sample[s]), DISCRETE_PT1_SET/5(T_Sample[s])
  Limit_n_Set/1(Out1) -> Gain2/1, SignalCollector/3(n_Set[rpm])
  n_Limit[rpm]/1 -> SignalCollector/1(n_Limit[rpm]), Limit_n_Set/2(In2)
  n[rpm]/1 -> Gain1/1
  Gain1/1 -> DISCRETE_PT1/2(In)
  Constant1/1 -> DISCRETE_PT1/1(Reset[0|1])
  Constant2/1 -> DISCRETE_PT1/3(K)
  DISCRETE_PT1/1(Out) -> PI_CONTROLLER/1(ActualValue), Gain3/1
  T_Filter[s]_n/1 -> DISCRETE_PT1/4(T[s])
  Gain2/1 -> PI_CONTROLLER/2(RefValue)
  Gain3/1 -> SignalCollector/2(n[rpm])
  n_Set[rpm]/1 -> DISCRETE_PT1_SET/2(In), Switch/1
  Constant3/1 -> DISCRETE_PT1_SET/4(T[s])
  Constant4/1 -> DISCRETE_PT1_SET/3(K)
  Constant5/1 -> DISCRETE_PT1_SET/1(Reset[0|1])
  DISCRETE_PT1_SET/1(Out) -> Switch/3
  Switch/1 -> Limit_n_Set/1(In1)
  switch_filter/1 -> Switch/2

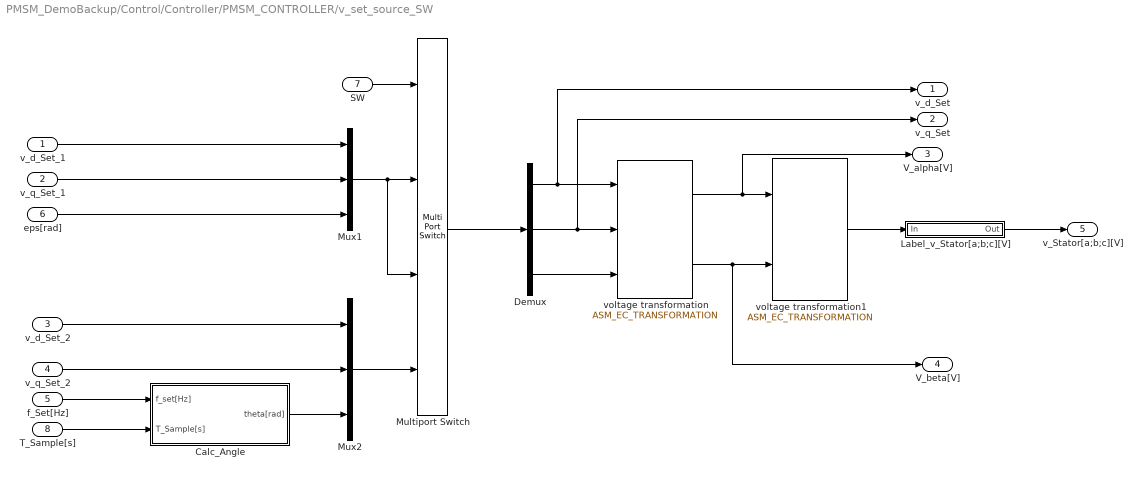
== system PMSM_DemoBackup/Control/Controller/PMSM_CONTROLLER/v_set_source_SW ==
  v_d_Set_1 : Inport
  v_q_Set_1 : Inport  Port=2
  v_d_Set_2 : Inport  Port=3
  v_q_Set_2 : Inport  Port=4
  f_Set[Hz] : Inport  Port=5
  eps[rad] : Inport  Port=6
  SW : Inport  Port=7
  T_Sample[s] : Inport  Port=8
  Calc_Angle : Subsystem
  Demux : Demux  Outputs=3
  Label_v_Stator[a;b;c][V] : Subsystem
  Multiport Switch : MultiPortSwitch
  Mux1 : Mux  Inputs=3
  Mux2 : Mux  Inputs=3
  voltage transformation : ASM_ElectricComponents_lib/Utils/ASM_EC_TRANSFORMATION  Description=version  transformation="d/q             -> alpha/beta  (inverse park transformation)"  compin=on  compout=on  zerocomp=off  interm=off  cossinvector=off  powrefframe=off  transffactor=1  transffactor_zero=1  ASMProperties=struct('Name','asm_ec_transformation','Version','1.0','Library','ASM_ElectricComponents_lib')
      settings: AttributesFormatString=inverse park transformation
  voltage transformation1 : ASM_ElectricComponents_lib/Utils/ASM_EC_TRANSFORMATION  Description=version  transformation="alpha/beta -> abc              (inverse clarke transformation)"  compin=on  compout=off  zerocomp=off  interm=off  cossinvector=off  powrefframe=off  transffactor=1  transffactor_zero=1  ASMProperties=struct('Name','asm_ec_transformation','Version','1.0','Library','ASM_ElectricComponents_lib')
      settings: AttributesFormatString=invers clark transformation
  v_d_Set : Outport  VectorParamsAs1DForOutWhenUnconnected=off
  v_q_Set : Outport  Port=2  VectorParamsAs1DForOutWhenUnconnected=off
  V_alpha[V] : Outport  Port=3  VectorParamsAs1DForOutWhenUnconnected=off
  V_beta[V] : Outport  Port=4  VectorParamsAs1DForOutWhenUnconnected=off
  v_Stator[a;b;c][V] : Outport  Port=5  VectorParamsAs1DForOutWhenUnconnected=off
  wires:
  SW/1 -> Multiport Switch/1
  Mux2/1 -> Multiport Switch/4
  Mux1/1 -> Multiport Switch/3, Multiport Switch/2
  Label_v_Stator[a;b;c][V]/1(Out) -> v_Stator[a;b;c][V]/1
  voltage transformation1/1 -> Label_v_Stator[a;b;c][V]/1(In)
  T_Sample[s]/1 -> Calc_Angle/2(T_Sample[s])
  v_d_Set_1/1 -> Mux1/1
  Demux/1 -> v_d_Set/1, voltage transformation/1
  Demux/2 -> v_q_Set/1, voltage transformation/2
  v_q_Set_1/1 -> Mux1/2
  v_d_Set_2/1 -> Mux2/1
  v_q_Set_2/1 -> Mux2/2
  eps[rad]/1 -> Mux1/3
  Demux/3 -> voltage transformation/3
  f_Set[Hz]/1 -> Calc_Angle/1(f_set[Hz])
  Calc_Angle/1(theta[rad]) -> Mux2/3
  Multiport Switch/1 -> Demux/1
  voltage transformation/1 -> voltage transformation1/1, V_alpha[V]/1
  voltage transformation/2 -> voltage transformation1/2, V_beta[V]/1

== system PMSM_DemoBackup/Control/Controller/SPACE_VECTOR_MODULATOR/Label_DutyCycle_HSD[a;b;c][0_1] ==
  In : Inport
  Bus Creator : BusCreator  Inputs=3
  Demux : Demux  Outputs=3
  Out : Outport  VectorParamsAs1DForOutWhenUnconnected=off
  wires:
  Demux/3 -> Bus Creator/3  "DutyCycle_c_HSD[0_1]"
  Demux/2 -> Bus Creator/2  "DutyCycle_b_HSD[0_1]"
  Demux/1 -> Bus Creator/1  "DutyCycle_a_HSD[0_1]"
  Bus Creator/1 -> Out/1  "DutyCycle_HSD[a;b;c][0_1]"
  In/1 -> Demux/1

== system PMSM_DemoBackup/Control/Controller/SPACE_VECTOR_MODULATOR/Label_DutyCycle_LSD[a;b;c][0_1] ==
  In : Inport
  Bus Creator : BusCreator  Inputs=3
  Demux : Demux  Outputs=3
  Out : Outport  VectorParamsAs1DForOutWhenUnconnected=off
  wires:
  In/1 -> Demux/1
  Bus Creator/1 -> Out/1  "DutyCycle_LSD[a;b;c][0_1]"
  Demux/1 -> Bus Creator/1  "DutyCycle_a_LSD[0_1]"
  Demux/2 -> Bus Creator/2  "DutyCycle_b_LSD[0_1]"
  Demux/3 -> Bus Creator/3  "DutyCycle_c_LSD[0_1]"

== system PMSM_DemoBackup/Control/Controller/SPACE_VECTOR_MODULATOR/SignalCollector ==
  DutyCycle_HSD[a;b;c][0_1] : Inport
  DutyCycle_LSD[a;b;c][0_1] : Inport  Port=2
  Bus Creator : BusCreator  Inputs=2
  SignalBus : Outport  VectorParamsAs1DForOutWhenUnconnected=off
  wires:
  Bus Creator/1 -> SignalBus/1  "SPACE_VECTOR_MODULATOR"
  DutyCycle_HSD[a;b;c][0_1]/1 -> Bus Creator/1  "DutyCycle_HSD[a;b;c][0_1]"
  DutyCycle_LSD[a;b;c][0_1]/1 -> Bus Creator/2  "DutyCycle_LSD[a;b;c][0_1]"

== system PMSM_DemoBackup/Control/Input/DISCRETE_PT1/discrete_Integrator_Init ==
  Reset[0|1] : Inport
  In : Inport  Port=2
  Initial : Inport  Port=3
  T_Sample[s] : Inport  Port=4
  Add : Sum  Inputs=+++
  Compare To Constant : simulink/Logic and Bit Operations/Compare To Constant  relop===  const=0  OutDataTypeStr=uint8  ZeroCross=off
  Constant1 : Constant  Value=0
  Constant2 : Constant  Value=0
  Logical Operator : Logic  Operator=OR  AllPortsSameDT=off  OutDataTypeStr=boolean
  Product : Product  RndMeth=Zero
  Saturation : simulink/Discontinuities/Saturation Dynamic  OutMin=[]  OutMax=[]  OutDataTypeStr=Inherit: Same as second input  OutDataType=sfix(16)  OutScaling=2^-10  DoSatur=off
  Switch1 : Switch  Threshold=0.5
  Switch2 : Switch  Threshold=0.5
  Unit Delay : UnitDelay  SampleTime=-1  HasFrameUpgradeWarning=on
  Unit Delay1 : UnitDelay  SampleTime=-1  HasFrameUpgradeWarning=on
  lower_limit : Constant  Value=lower_limit.v
  "only_rising_edge " : Subsystem
  upper_limit : Constant  Value=upper_limit.v
  Out : Outport  VectorParamsAs1DForOutWhenUnconnected=off
  wires:
  Compare To Constant/1 -> Logical Operator/1
  Logical Operator/1 -> Switch1/2
  Unit Delay1/1 -> Compare To Constant/1
  "only_rising_edge "/1(Out1) -> Switch2/2, Logical Operator/2
  Constant1/1 -> Switch1/3
  Initial/1 -> Switch1/1
  Switch1/1 -> Add/1
  Unit Delay/1 -> Switch2/3
  Switch2/1 -> Add/3
  Constant2/1 -> Switch2/1
  In/1 -> Product/2
  Reset[0|1]/1 -> "only_rising_edge "/1(In1)
  Product/1 -> Add/2
  T_Sample[s]/1 -> Unit Delay1/1, Product/1
  Add/1 -> Saturation/2
  Saturation/1 -> Out/1, Unit Delay/1
  upper_limit/1 -> Saturation/1
  lower_limit/1 -> Saturation/3

== system PMSM_DemoBackup/RTI Data/RTI Data Store/RTI Data Store/RTI Data Store ==
  RTI Data Store : Subsystem  mask(RTI_DATA_STORE){}
      mask help:
      | RTI Data Store Block. This block is used by RTI to store internal model dependent data. Deleting this block will result in data loss.
      |
      | NEVER DELETE, COPY, OR MODIFY THIS BLOCK!
      mask Help:
      | RTI Data Store Block. This block is used by RTI to store internal model dependent data. Deleting this block will result in data loss.
      | 
      | NEVER DELETE, COPY, OR MODIFY THIS BLOCK!
      mask Display: text(0.5, 0.5, ' ', 'HorizontalAlignment', 'center');

== system PMSM_DemoBackup/Control/Controller/PMSM_CONTROLLER/angle_calculation/Lim[0...2*pi] ==
  theta_unlim : Inport
  Constant2 : Constant  Value=2*pi
  Math Function1 : Math  Operator=mod  SignedPower=on  SaturateOnIntegerOverflow=on
  theta_lim : Outport  VectorParamsAs1DForOutWhenUnconnected=off
  wires:
  Constant2/1 -> Math Function1/2
  Math Function1/1 -> theta_lim/1
  theta_unlim/1 -> Math Function1/1

== system PMSM_DemoBackup/Control/Controller/PMSM_CONTROLLER/current_controller/DISCRETE_PT1 ==
  Reset[0|1] : Inport
  In : Inport  Port=2
  K : Inport  Port=3
  T[s] : Inport  Port=4
  T_Sample[s] : Inport  Port=5
  1|FilterTime : Product  Inputs=*/  InputSameDT=on  SaturateOnIntegerOverflow=on  OutDataTypeStr=Inherit: Same as first input
  Proportional : Product  Inputs=**  InputSameDT=on  SaturateOnIntegerOverflow=on  OutDataTypeStr=Inherit: Same as first input
  Sum : Sum  Inputs=-+|  InputSameDT=on  SaturateOnIntegerOverflow=on  OutDataTypeStr=Inherit: Same as first input
  Unit Delay : UnitDelay  SampleTime=-1  HasFrameUpgradeWarning=on
  discrete_Integrator_Init : Subsystem  mask(DISCRETE_INTEGRATOR){upper_limit=upper_limit_int, lower_limit=lower_limit_int, ASMProperties=struct('Name','discrete_integrator','Version','1.0','Library','ASM_ElectricComponents_lib')}
      mask prompts: upper_limit "upper limit"; lower_limit "lower limit"
      mask help: (c) Copyright 2007, dSPACE GmbH. All rights reserved.
      mask Help: eval(['asm_modelhelp(gcbh)'])
  zero : Constant  Value=0  SampleTime=-1
  Out : Outport  VectorParamsAs1DForOutWhenUnconnected=off
  wires:
  In/1 -> Proportional/1
  Sum/1 -> discrete_Integrator_Init/2(In)
  K/1 -> Proportional/2
  Proportional/1 -> Sum/2
  discrete_Integrator_Init/1(Out) -> 1|FilterTime/1
  1|FilterTime/1 -> Out/1, Unit Delay/1
  Unit Delay/1 -> Sum/1
  T[s]/1 -> 1|FilterTime/2
  Reset[0|1]/1 -> discrete_Integrator_Init/1(Reset[0|1])
  T_Sample[s]/1 -> discrete_Integrator_Init/4(T_Sample[s])
  zero/1 -> discrete_Integrator_Init/3(Initial)

== system PMSM_DemoBackup/Control/Controller/PMSM_CONTROLLER/current_controller/DISCRETE_PT2 ==
  Reset[0|1] : Inport
  In : Inport  Port=2
  K : Inport  Port=3
  T[s] : Inport  Port=4
  T_Sample[s] : Inport  Port=5
  1|FilterTime : Product  Inputs=*/  InputSameDT=on  SaturateOnIntegerOverflow=on  OutDataTypeStr=Inherit: Same as first input
  Proportional : Product  Inputs=**  InputSameDT=on  SaturateOnIntegerOverflow=on  OutDataTypeStr=Inherit: Same as first input
  Sum : Sum  Inputs=-+|  InputSameDT=on  SaturateOnIntegerOverflow=on  OutDataTypeStr=Inherit: Same as first input
  Unit Delay : UnitDelay  SampleTime=-1  HasFrameUpgradeWarning=on
  discrete_Integrator_Init : Subsystem  mask(DISCRETE_INTEGRATOR){upper_limit=upper_limit_int, lower_limit=lower_limit_int, ASMProperties=struct('Name','discrete_integrator','Version','1.0','Library','ASM_ElectricComponents_lib')}
      mask prompts: upper_limit "upper limit"; lower_limit "lower limit"
      mask help: (c) Copyright 2007, dSPACE GmbH. All rights reserved.
      mask Help: eval(['asm_modelhelp(gcbh)'])
  zero : Constant  Value=0  SampleTime=-1
  Out : Outport  VectorParamsAs1DForOutWhenUnconnected=off
  wires:
  zero/1 -> discrete_Integrator_Init/3(Initial)
  T_Sample[s]/1 -> discrete_Integrator_Init/4(T_Sample[s])
  Reset[0|1]/1 -> discrete_Integrator_Init/1(Reset[0|1])
  T[s]/1 -> 1|FilterTime/2
  Unit Delay/1 -> Sum/1
  1|FilterTime/1 -> Unit Delay/1, Out/1
  discrete_Integrator_Init/1(Out) -> 1|FilterTime/1
  Proportional/1 -> Sum/2
  K/1 -> Proportional/2
  Sum/1 -> discrete_Integrator_Init/2(In)
  In/1 -> Proportional/1

== system PMSM_DemoBackup/Control/Controller/PMSM_CONTROLLER/current_controller/PI_CONTROLLER_id ==
  ActualValue : Inport
  RefValue : Inport  Port=2
  Kp : Inport  Port=3
  Ki : Inport  Port=4
  y_limited : Inport  Port=5
  T_Sample[s] : Inport  Port=6
  Product : Product  RndMeth=Zero
  Product1 : Product  RndMeth=Zero
  Product2 : Product  RndMeth=Zero
  Sum : Sum  Inputs=+++  SaturateOnIntegerOverflow=on
  Sum1 : Sum  Inputs=+-  SaturateOnIntegerOverflow=on
  Sum2 : Sum  Inputs=-|+  SaturateOnIntegerOverflow=on
  Unit Delay : UnitDelay  SampleTime=-1  HasFrameUpgradeWarning=on
  y : Outport  VectorParamsAs1DForOutWhenUnconnected=off
  wires:
  T_Sample[s]/1 -> Product/2
  Sum2/1 -> Unit Delay/1
  Unit Delay/1 -> Sum/3
  Product2/1 -> Product/1
  Sum/1 -> y/1
  Product/1 -> Sum/2  "integral"
  Product1/1 -> Sum2/1, Sum/1
  ActualValue/1 -> Sum1/2
  RefValue/1 -> Sum1/1
  Sum1/1 -> Product1/2, Product2/2  "error"
  y_limited/1 -> Sum2/2
  Kp/1 -> Product1/1
  Ki/1 -> Product2/1

== system PMSM_DemoBackup/Control/Controller/PMSM_CONTROLLER/current_controller/PI_CONTROLLER_iq ==
  ActualValue : Inport
  RefValue : Inport  Port=2
  Kp : Inport  Port=3
  Ki : Inport  Port=4
  y_limited : Inport  Port=5
  T_Sample[s] : Inport  Port=6
  Product : Product  RndMeth=Zero
  Product1 : Product  RndMeth=Zero
  Product2 : Product  RndMeth=Zero
  Sum : Sum  Inputs=+++  SaturateOnIntegerOverflow=on
  Sum1 : Sum  Inputs=+-  SaturateOnIntegerOverflow=on
  Sum2 : Sum  Inputs=-|+  SaturateOnIntegerOverflow=on
  Unit Delay : UnitDelay  SampleTime=-1  HasFrameUpgradeWarning=on
  y : Outport  VectorParamsAs1DForOutWhenUnconnected=off
  wires:
  T_Sample[s]/1 -> Product/2
  Sum2/1 -> Unit Delay/1
  Unit Delay/1 -> Sum/3
  Product2/1 -> Product/1
  Sum/1 -> y/1
  Product/1 -> Sum/2  "integral"
  Product1/1 -> Sum2/1, Sum/1
  ActualValue/1 -> Sum1/2
  RefValue/1 -> Sum1/1
  Sum1/1 -> Product1/2, Product2/2  "error"
  y_limited/1 -> Sum2/2
  Kp/1 -> Product1/1
  Ki/1 -> Product2/1

== system PMSM_DemoBackup/Control/Controller/PMSM_CONTROLLER/current_controller/SignalCollector ==
  i_alpha[A] : Inport
  i_beta[A] : Inport  Port=2
  I_d[A] : Inport  Port=3
  I_d_Set[A] : Inport  Port=4
  I_q_Set[A] : Inport  Port=5
  I_q[A] : Inport  Port=6
  V_d_Ctrl_lim[V] : Inport  Port=7
  V_d_Set[V] : Inport  Port=8
  V_q_Set[V] : Inport  Port=9
  V_d_Ctrl_unlim[V] : Inport  Port=10
  V_q_Ctrl_unlim[V] : Inport  Port=11
  V_q_Ctrl_lim[V] : Inport  Port=12
  Bus Creator : BusCreator  Inputs=12
  ASMSignalBus : Outport  VectorParamsAs1DForOutWhenUnconnected=off
  wires:
  V_q_Ctrl_lim[V]/1 -> Bus Creator/10  "V_q_Ctrl_lim[V]"
  V_d_Ctrl_lim[V]/1 -> Bus Creator/9  "V_d_Ctrl_lim[V]"
  V_q_Set[V]/1 -> Bus Creator/8  "V_q_Set[V]"
  V_d_Set[V]/1 -> Bus Creator/7  "V_d_Set[V]"
  V_q_Ctrl_unlim[V]/1 -> Bus Creator/6  "V_q_Ctrl_unlim[V]"
  V_d_Ctrl_unlim[V]/1 -> Bus Creator/5  "V_d_Ctrl_unlim[V]"
  I_q_Set[A]/1 -> Bus Creator/4  "I_q_Set[A]"
  I_d_Set[A]/1 -> Bus Creator/3  "I_d_Set[A]"
  I_q[A]/1 -> Bus Creator/2  "I_q[A]"
  I_d[A]/1 -> Bus Creator/1  "I_d[A]"
  Bus Creator/1 -> ASMSignalBus/1  "CURRENT_CONTROLLER"
  i_alpha[A]/1 -> Bus Creator/11  "i_alpha[A]"
  i_beta[A]/1 -> Bus Creator/12  "i_beta[A]"

== system PMSM_DemoBackup/Control/Controller/PMSM_CONTROLLER/current_controller/current transformation ==
  in1 : Inport
  in2 : Inport  Port=2
  demux : Demux  Outputs=2
      settings: DisplayOption=none
  mux : Mux  Inputs=2
  transf : Subsystem
      settings: AttributesFormatString=clarkepark
  out1 : Outport  VectorParamsAs1DForOutWhenUnconnected=off
  out2 : Outport  Port=2  VectorParamsAs1DForOutWhenUnconnected=off
  wires:
  mux/1 -> transf/1(in)
  in1/1 -> mux/1
  in2/1 -> mux/2
  transf/1(out) -> demux/1
  demux/1 -> out1/1
  demux/2 -> out2/1

== system PMSM_DemoBackup/Control/Controller/PMSM_CONTROLLER/current_controller/current_transformation_disp ==
  in1 : Inport
  demux : Demux  Outputs=2
      settings: DisplayOption=none
  transf : Subsystem
      settings: AttributesFormatString=clarke
  out1 : Outport  VectorParamsAs1DForOutWhenUnconnected=off
  out2 : Outport  Port=2  VectorParamsAs1DForOutWhenUnconnected=off
  wires:
  in1/1 -> transf/1(in)
  transf/1(out) -> demux/1
  demux/1 -> out1/1
  demux/2 -> out2/1
